simulink model "PIDTuningOpenLoop"  (R2017a)
settings: Solver=VariableStepAuto  StartTime=0.0  StopTime=duur  RelTol=1e-3  EnableMultiTasking=on
values from neighbouring files (symbols this model uses):
  K1 = 1    [PIDTuning.m]
  K2 = 3    [PIDTuning.m]    (also in margin.m)
  Km = 1    [PIDTuning.m]    (also in margin.m)
  tau1 = 2    [PIDTuning.m]    (also in PIDcontroller.m; margin.m)
  tau2 = 6    [PIDTuning.m]    (also in PIDcontroller.m; margin.m)
  taum = 0.2    [PIDTuning.m]    (also in margin.m)
settings Model: Creator=wrquaghe  LastModifiedBy=geert
settings DataIOCC: LimitDataPoints=on
settings OptimizationCC: LifeSpan=inf
settings DebuggingCC: AllowSymbolicDim=off  SFUnexpectedBacktrackingDiag=warning  SFNoUnconditionalDefaultTransitionDiag=warning  SFExecutionAtInitializationDiag=none
settings ModelReferenceCC: PropagateSignalLabelsOutOfModel=off
settings GRTTargetCC: TargetLangStandard=C89/C90 (ANSI)
settings ConfigComp: CovMetricSettings=dw  CovHtmlReporting=on  CovSaveCumulativeToWorkspaceVar=on  CovSaveSingleToWorkspaceVar=on  CovExternalEMLEnable=off

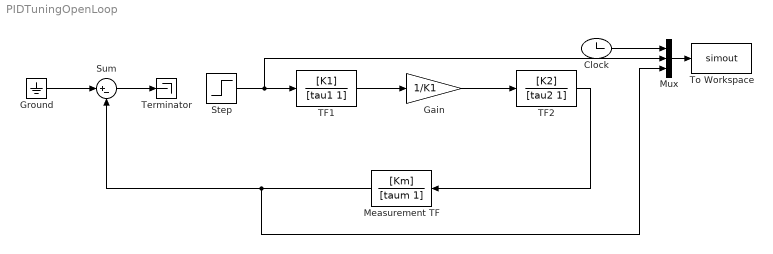
== system PIDTuningOpenLoop ==
  Clock : Clock
  Gain : Gain  Gain=1/K1
  Ground : Ground
  Measurement TF : TransferFcn  Numerator=[Km]  Denominator=[taum 1]
  Mux : Mux  Inputs=3
  Step : Step  Time=0  SampleTime=0
  Sum : Sum  Inputs=|+-
  TF1 : TransferFcn  Numerator=[K1]  Denominator=[tau1 1]
  TF2 : TransferFcn  Numerator=[K2]  Denominator=[tau2 1]
  Terminator : Terminator
  To Workspace : ToWorkspace  VariableName=simout  SampleTime=1
  wires:
  Ground/1 -> Sum/1
  Sum/1 -> Terminator/1
  TF1/1 -> Gain/1
  Gain/1 -> TF2/1
  TF2/1 -> Measurement TF/1
  Measurement TF/1 -> Mux/3, Sum/2
  Step/1 -> Mux/2, TF1/1
  Clock/1 -> Mux/1
  Mux/1 -> To Workspace/1
